simulink model "Nonlinear_RBD"  (R2023b)
settings: Solver=ode4  StartTime=0  StopTime=tfinal  FixedStep=dt  RelTol=1e-3
values from neighbouring files (symbols this model uses):
  F_gravity_0 = mass * gravity * [sin(states_0(8));                                 -cos(states_0(8)) * sin(states_0(7));                                 -cos(states_0(8)) * cos(states_0(7))]    [main_code.m]    (also in untitled4.m; untitled5.m)
  gravity = [-Mass*g*sin(Current_States(8)) ... (first row only)    [Airframe_Model.m]    (also in main_code.m = aircraft_data(52); untitled4.m = aircraft_data(52); untitled5.m = aircraft_data(52))
  Ixx = aircraft_data(53)    [main_code.m]    (also in untitled4.m; untitled5.m)
  Iyy = aircraft_data(54)    [main_code.m]    (also in untitled4.m; untitled5.m)
  Izz = aircraft_data(55)    [main_code.m]    (also in untitled4.m; untitled5.m)
  M_0 = [0; 0; 0]    [main_code.m]    (also in untitled4.m; untitled5.m)
  mass = aircraft_data(51)    [main_code.m]    (also in untitled4.m; untitled5.m)
  Matrix_controls = [0, Xde, Xdth, 0 ... (first row only)    [main_code.m]    (also in untitled4.m)
  Matrix_states = [Xu, 0, Xw, 0, 0, 0, 0 ... (first row only)    [main_code.m]    (also in untitled4.m)
  p0 = states_0(4)    [main_code.m]    (also in untitled4.m; untitled5.m = Vomega_0(1))
  phi0 = states_0(7)    [main_code.m]    (also in untitled4.m)
  psi0 = states_0(9)    [main_code.m]    (also in untitled4.m)
  q0 = states_0(5)    [main_code.m]    (also in untitled4.m; untitled5.m = Vomega_0(2))
  r0 = states_0(6)    [main_code.m]    (also in untitled4.m; untitled5.m = Vomega_0(3))
  states_0 = aircraft_data(4:15)    [main_code.m]    (also in untitled4.m; untitled5.m)
  theta0 = states_0(8)    [main_code.m]    (also in untitled4.m)
  u0 = states_0(1)    [main_code.m]    (also in untitled4.m; untitled5.m = Vb_0(1))
  v0 = states_0(2)    [main_code.m]    (also in untitled4.m; untitled5.m = Vb_0(2))
  w0 = states_0(3)    [main_code.m]    (also in untitled4.m; untitled5.m = Vb_0(3))
  x0 = states_0(10)    [main_code.m]    (also in untitled4.m)
  y0 = states_0(11)    [main_code.m]    (also in untitled4.m)
  z0 = states_0(12)    [main_code.m]    (also in untitled4.m)
libraries: dspsigops x2, shared6dof x1, aerolibasang x1
settings Model: Creator=Ahmed Raamadan  LastModifiedBy=Ahmed Raamadan

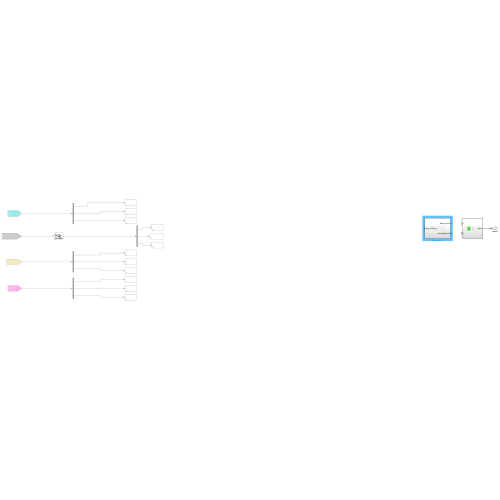
[thumbnail: Simulink's stored preview of the top-level diagram]
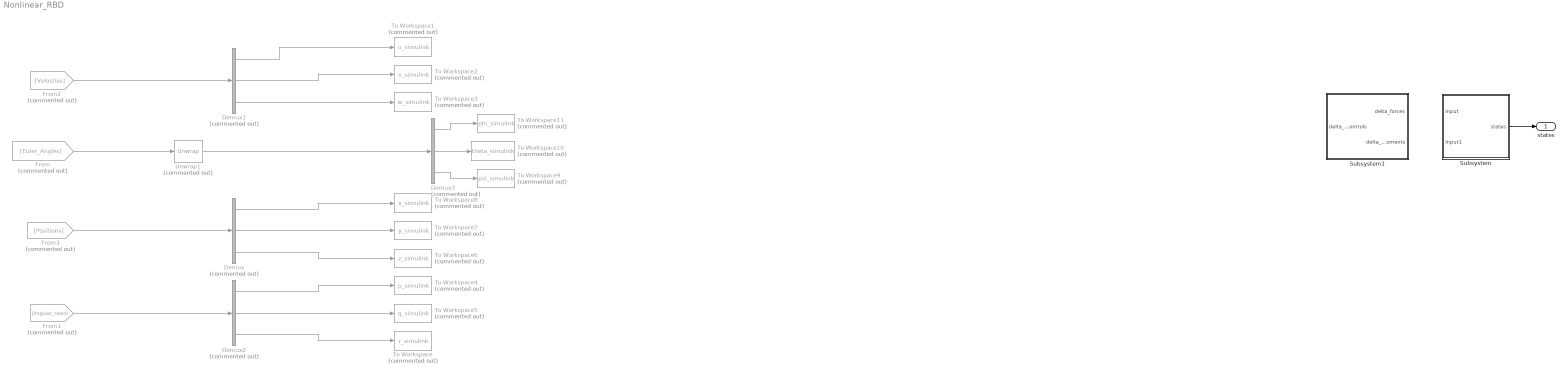
== system Nonlinear_RBD ==
  Demux{,1..3} (4 alike) : Demux  Commented=on  Outputs=3
  From : From  Commented=on  GotoTag=Euler_Angles
  From1 : From  Commented=on  GotoTag=Angular_rates
  From2 : From  Commented=on  GotoTag=Velosties
  From3 : From  Commented=on  GotoTag=Positions
  Subsystem : Subsystem
  Subsystem1 : Subsystem
  To Workspace : ToWorkspace  Commented=on  VariableName=r_simulink  SaveFormat=Timeseries  SampleTime=-1
  To Workspace1 : ToWorkspace  Commented=on  VariableName=u_simulink  SaveFormat=Timeseries  SampleTime=-1
  To Workspace10 : ToWorkspace  Commented=on  VariableName=theta_simulink  SaveFormat=Timeseries  SampleTime=-1
  To Workspace11 : ToWorkspace  Commented=on  VariableName=phi_simulink  SaveFormat=Timeseries  SampleTime=-1
  To Workspace2 : ToWorkspace  Commented=on  VariableName=v_simulink  SaveFormat=Timeseries  SampleTime=-1
  To Workspace3 : ToWorkspace  Commented=on  VariableName=w_simulink  SaveFormat=Timeseries  SampleTime=-1
  To Workspace4 : ToWorkspace  Commented=on  VariableName=p_simulink  SaveFormat=Timeseries  SampleTime=-1
  To Workspace5 : ToWorkspace  Commented=on  VariableName=q_simulink  SaveFormat=Timeseries  SampleTime=-1
  To Workspace6 : ToWorkspace  Commented=on  VariableName=z_simulink  SaveFormat=Timeseries  SampleTime=-1
  To Workspace7 : ToWorkspace  Commented=on  VariableName=y_simulink  SaveFormat=Timeseries  SampleTime=-1
  To Workspace8 : ToWorkspace  Commented=on  VariableName=x_simulink  SaveFormat=Timeseries  SampleTime=-1
  To Workspace9 : ToWorkspace  Commented=on  VariableName=psi_simulink  SaveFormat=Timeseries  SampleTime=-1
  Unwrap1 : dspsigops/Unwrap  Commented=on  tol=pi  running=off
  states : Outport
  wires:
  From/1 -> Unwrap1/1
  From2/1 -> Demux1/1
  Demux1/1 -> To Workspace1/1
  From3/1 -> Demux/1
  From1/1 -> Demux2/1
  Demux3/2 -> To Workspace10/1
  Demux1/3 -> To Workspace3/1
  Demux/1 -> To Workspace8/1
  Demux2/1 -> To Workspace4/1
  Demux/2 -> To Workspace7/1
  Demux1/2 -> To Workspace2/1
  Unwrap1/1 -> Demux3/1
  Demux/3 -> To Workspace6/1
  Demux2/2 -> To Workspace5/1
  Demux2/3 -> To Workspace/1
  Demux3/3 -> To Workspace9/1
  Demux3/1 -> To Workspace11/1
  Subsystem/1(states) -> states/1

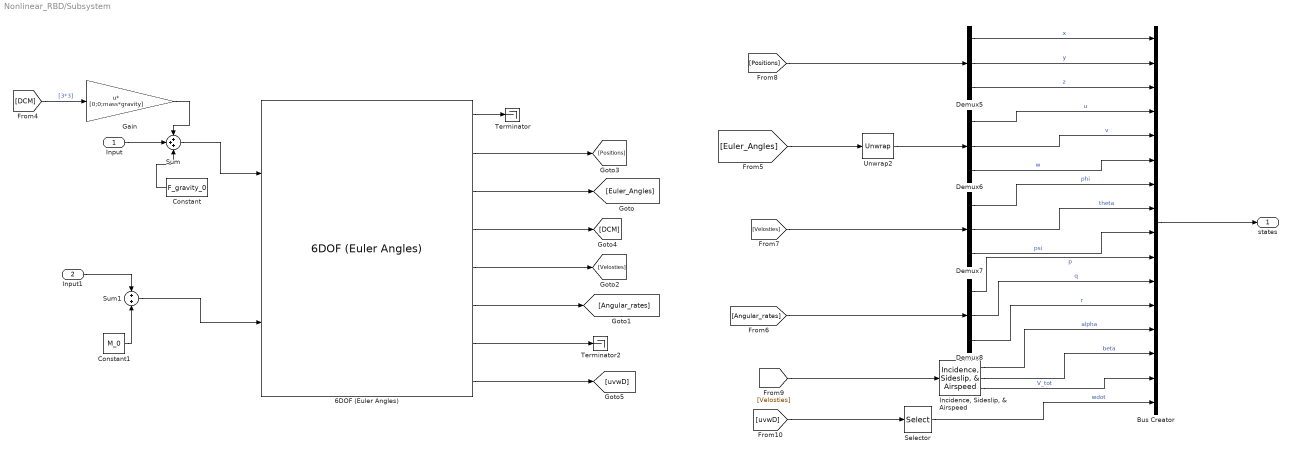
== system Nonlinear_RBD/Subsystem ==
  Input : Inport
  Input1 : Inport  Port=2
  6DOF (Euler Angles) : shared6dof/6DOF (Euler Angles)  units=English (Velocity in ft/s)  mtype=Fixed  rep=Euler Angles  xme_0=[x0 y0 z0]  Vm_0=[u0 v0 w0]  eul_0=[phi0 theta0 psi0]  pm_0=[p0 q0 r0]  mass_0=mass  mass_e=0.5  mass_f=2.0  inertia=Inertia  inertia_e=eye(3)  inertia_f=2*eye(3)  k_quat=1.0  vre_flag=on  abi_flag=off  aMode=0  xme_statename=''  Vm_statename=''  eul_statename=''  quat_statename=''  pm_statename=''  mass_statename=''
  Bus Creator : BusCreator  Inputs=16
  Constant : Constant  Value=F_gravity_0
  Constant1 : Constant  Value=M_0
  Demux{5..8} (4 alike) : Demux  Outputs=3
  Gain : Gain  Gain=[0;0;mass*gravity]  Multiplication=Matrix(u*K)
  "Incidence, Sideslip, & Airspeed" : aerolibasang/Incidence, Sideslip, & Airspeed
  Selector : Selector  InputPortWidth=3  IndexOptions=Index vector (dialog)  Indices=[3]  OutputSizes=1
  Sum : Sum  Inputs=+++
  Sum1 : Sum
  Terminator : Terminator
  Terminator2 : Terminator
  Unwrap2 : dspsigops/Unwrap  tol=pi  running=off
  states : Outport
  wires:
  Demux6/3 -> Bus Creator/6  "w"
  Unwrap2/1 -> Demux6/1
  Selector/1 -> Bus Creator/16  "wdot"
  Demux6/1 -> Bus Creator/4  "u"
  6DOF (Euler Angles)/3 -> [Euler_Angles]
  6DOF (Euler Angles)/5 -> [Velosties]
  [Angular_rates] -> Demux8/1
  "Incidence, Sideslip, & Airspeed"/1 -> Bus Creator/13  "alpha"
  [Euler_Angles] -> Unwrap2/1
  [DCM] -> Gain/1  "[3*3]"
  6DOF (Euler Angles)/4 -> [DCM]
  Demux8/2 -> Bus Creator/11  "q"
  Demux8/1 -> Bus Creator/10  "p"
  Sum/1 -> 6DOF (Euler Angles)/1
  "Incidence, Sideslip, & Airspeed"/2 -> Bus Creator/14  "beta"
  "Incidence, Sideslip, & Airspeed"/3 -> Bus Creator/15  "V_tot"
  Sum1/1 -> 6DOF (Euler Angles)/2
  Constant/1 -> Sum/3
  [Velosties] -> "Incidence, Sideslip, & Airspeed"/1
  6DOF (Euler Angles)/1 -> Terminator/1
  6DOF (Euler Angles)/7 -> Terminator2/1
  Demux8/3 -> Bus Creator/12  "r"
  Constant1/1 -> Sum1/2
  Demux6/2 -> Bus Creator/5  "v"
  [uvwD] -> Selector/1
  Gain/1 -> Sum/1
  Bus Creator/1 -> states/1
  Demux7/2 -> Bus Creator/8  "theta"
  6DOF (Euler Angles)/2 -> [Positions]
  6DOF (Euler Angles)/6 -> [Angular_rates]
  Demux5/2 -> Bus Creator/2  "y"
  6DOF (Euler Angles)/8 -> [uvwD]
  [Velosties] -> Demux7/1
  Demux7/3 -> Bus Creator/9  "psi"
  Demux7/1 -> Bus Creator/7  "phi"
  Demux5/3 -> Bus Creator/3  "z"
  Demux5/1 -> Bus Creator/1  "x"
  [Positions] -> Demux5/1
  Input/1 -> Sum/2
  Input1/1 -> Sum1/1

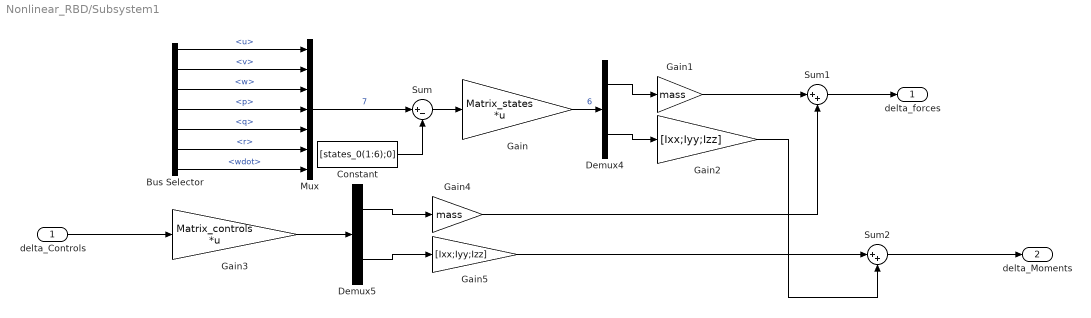
== system Nonlinear_RBD/Subsystem1 ==
  delta_Controls : Inport
  Bus Selector : BusSelector  OutputSignals=u,v,w,p,q,r,wdot
  Constant : Constant  Value=[states_0(1:6);0]  SampleTime=-1
  Demux4 : Demux  Outputs=2
  Demux5 : Demux  Outputs=2
  Gain : Gain  Gain=Matrix_states  Multiplication=Matrix(K*u)
  Gain1 : Gain  Gain=mass
  Gain2 : Gain  Gain=[Ixx;Iyy;Izz]
  Gain3 : Gain  Gain=Matrix_controls  Multiplication=Matrix(K*u)
  Gain4 : Gain  Gain=mass
  Gain5 : Gain  Gain=[Ixx;Iyy;Izz]
  Mux : Mux  Inputs=7
  Sum : Sum  Inputs=|+-
  Sum1 : Sum  Inputs=|++
  Sum2 : Sum  Inputs=|++
  delta_forces : Outport
  delta_Moments : Outport  Port=2
  wires:
  Gain3/1 -> Demux5/1
  Bus Selector/4 -> Mux/4  "<p>"
  Bus Selector/1 -> Mux/1  "<u>"
  Mux/1 -> Sum/1  "7"
  delta_Controls/1 -> Gain3/1
  Bus Selector/2 -> Mux/2  "<v>"
  Sum2/1 -> delta_Moments/1
  Demux5/2 -> Gain5/1
  Sum/1 -> Gain/1
  Bus Selector/3 -> Mux/3  "<w>"
  Demux4/1 -> Gain1/1
  Gain1/1 -> Sum1/1
  Constant/1 -> Sum/2
  Demux4/2 -> Gain2/1
  Demux5/1 -> Gain4/1
  Gain/1 -> Demux4/1  "6"
  Gain5/1 -> Sum2/1
  Gain4/1 -> Sum1/2
  Sum1/1 -> delta_forces/1
  Bus Selector/5 -> Mux/5  "<q>"
  Bus Selector/7 -> Mux/7  "<wdot>"
  Gain2/1 -> Sum2/2
  Bus Selector/6 -> Mux/6  "<r>"
